simulink model "case6"  (R2024b)
settings: Solver=FixedStepAuto  StartTime=0  StopTime=1  FixedStep=1e-7  RelTol=1e-3
values from neighbouring files (symbols this model uses):
  SG_D_1_D = 0.01056    [IEEE9_case_parameters.m]    (also in case1_parameters.m; case2_parameters.m; case3_parameters.m; case4_parameters.m)
  SG_D_1_EnableSaturation = 0    [IEEE9_case_parameters.m]    (also in case1_parameters.m; case2_parameters.m; case3_parameters.m; case4_parameters.m)
  SG_D_1_f0 = 60    [IEEE9_case_parameters.m]    (also in case1_parameters.m; case2_parameters.m; case3_parameters.m; case4_parameters.m)
  SG_D_1_H = 7.5    [IEEE9_case_parameters.m]    (also in case1_parameters.m; case2_parameters.m; case3_parameters.m; case4_parameters.m)
  SG_D_1_K_A = 20    [IEEE9_case_parameters.m]    (also in case1_parameters.m; case2_parameters.m; case3_parameters.m; case4_parameters.m)
  SG_D_1_K_E = 1.000000e+1    (= 10)    [IEEE9_case_parameters.m]    (also in case1_parameters.m; case2_parameters.m; case3_parameters.m; case4_parameters.m)
  SG_D_1_K_F = 2.363    [IEEE9_case_parameters.m]    (also in case1_parameters.m; case2_parameters.m; case3_parameters.m; case4_parameters.m)
  SG_D_1_K_s = 0.5    [IEEE9_case_parameters.m]    (also in case1_parameters.m = 5; case2_parameters.m = 5; case3_parameters.m = 5; case4_parameters.m = 5)
  SG_D_1_R_a = 0.001088    [IEEE9_case_parameters.m]    (also in case1_parameters.m; case2_parameters.m; case3_parameters.m; case4_parameters.m)
  SG_D_1_S_A = 1    [IEEE9_case_parameters.m]    (also in case1_parameters.m; case2_parameters.m; case3_parameters.m; case4_parameters.m)
  SG_D_1_S_B = 0.103    [IEEE9_case_parameters.m]    (also in case1_parameters.m; case2_parameters.m; case3_parameters.m; case4_parameters.m)
  SG_D_1_S_N = 10.659857    [IEEE9_case_parameters.m]    (also in case1_parameters.m; case2_parameters.m; case3_parameters.m; case4_parameters.m)
  SG_D_1_SpeedPara = 200    [IEEE9_case_parameters.m]    (also in case1_parameters.m; case2_parameters.m; case3_parameters.m; case4_parameters.m)
  SG_D_1_T_0 = 0.720173    [IEEE9_case_parameters.m]    (also in case1_parameters.m = 0.755522; case2_parameters.m = 0.808931; case3_parameters.m = 0.869402; case4_parameters.m = 0.729316)
  SG_D_1_T_1 = 0.3    [IEEE9_case_parameters.m]    (also in case1_parameters.m; case2_parameters.m; case3_parameters.m; case4_parameters.m)
  SG_D_1_T_2 = 0.05    [IEEE9_case_parameters.m]    (also in case1_parameters.m; case2_parameters.m; case3_parameters.m; case4_parameters.m)
  SG_D_1_T_3 = 0.02    [IEEE9_case_parameters.m]    (also in case1_parameters.m; case2_parameters.m; case3_parameters.m; case4_parameters.m)
  SG_D_1_T_4 = 0.005    [IEEE9_case_parameters.m]    (also in case1_parameters.m; case2_parameters.m; case3_parameters.m; case4_parameters.m)
  SG_D_1_T_A = 0.02    [IEEE9_case_parameters.m]    (also in case1_parameters.m; case2_parameters.m; case3_parameters.m; case4_parameters.m)
  SG_D_1_T_dd = 8.000000e+0    (= 8)    [IEEE9_case_parameters.m]    (also in case1_parameters.m; case2_parameters.m; case3_parameters.m; case4_parameters.m)
  SG_D_1_T_ddd = 0.04    [IEEE9_case_parameters.m]    (also in case1_parameters.m; case2_parameters.m; case3_parameters.m; case4_parameters.m)
  SG_D_1_T_E = 0.314    [IEEE9_case_parameters.m]    (also in case1_parameters.m; case2_parameters.m; case3_parameters.m; case4_parameters.m)
  SG_D_1_T_F = 0.35    [IEEE9_case_parameters.m]    (also in case1_parameters.m; case2_parameters.m; case3_parameters.m; case4_parameters.m)
  SG_D_1_T_qd = 0.8    [IEEE9_case_parameters.m]    (also in case1_parameters.m; case2_parameters.m; case3_parameters.m; case4_parameters.m)
  SG_D_1_T_qdd = 0.02    [IEEE9_case_parameters.m]    (also in case1_parameters.m; case2_parameters.m; case3_parameters.m; case4_parameters.m)
  SG_D_1_T_speed = 0.1    [IEEE9_case_parameters.m]    (also in case1_parameters.m = 200; case2_parameters.m = 200; case3_parameters.m = 200; case4_parameters.m = 200)
  SG_D_1_T_w = 0.5    [IEEE9_case_parameters.m]    (also in case1_parameters.m; case2_parameters.m; case3_parameters.m; case4_parameters.m)
  SG_D_1_V_ref = 1.990276    [IEEE9_case_parameters.m]    (also in case1_parameters.m = 2.042296; case2_parameters.m = 2.051388; case3_parameters.m = 2.089584; case4_parameters.m = 2.01845)
  SG_D_1_w_ref = 376.991118    [IEEE9_case_parameters.m]    (also in case1_parameters.m; case2_parameters.m; case3_parameters.m; case4_parameters.m)
  SG_D_1_wb = 6.000000e+1    (= 60)    [IEEE9_case_parameters.m]    (also in case1_parameters.m; case2_parameters.m; case3_parameters.m; case4_parameters.m)
  SG_D_1_x_d = 1.9    [IEEE9_case_parameters.m]    (also in case1_parameters.m; case2_parameters.m; case3_parameters.m; case4_parameters.m)
  SG_D_1_x_dd = 0.302    [IEEE9_case_parameters.m]    (also in case1_parameters.m; case2_parameters.m; case3_parameters.m; case4_parameters.m)
  SG_D_1_x_ddd = 0.204    [IEEE9_case_parameters.m]    (also in case1_parameters.m; case2_parameters.m; case3_parameters.m; case4_parameters.m)
  SG_D_1_x_l = 0.05    [IEEE9_case_parameters.m]    (also in case1_parameters.m; case2_parameters.m; case3_parameters.m; case4_parameters.m)
  SG_D_1_x_q = 1.3    [IEEE9_case_parameters.m]    (also in case1_parameters.m; case2_parameters.m; case3_parameters.m; case4_parameters.m)
  SG_D_1_x_qd = 0.5    [IEEE9_case_parameters.m]    (also in case1_parameters.m; case2_parameters.m; case3_parameters.m; case4_parameters.m)
  SG_D_1_x_qdd = 0.3    [IEEE9_case_parameters.m]    (also in case1_parameters.m; case2_parameters.m; case3_parameters.m; case4_parameters.m)
  SG_D_2_D = 0.02    [IEEE9_case_parameters.m]    (also in case1_parameters.m; case2_parameters.m; case3_parameters.m; case4_parameters.m)
  SG_D_2_EnableSaturation = 0    [IEEE9_case_parameters.m]    (also in case1_parameters.m; case2_parameters.m; case3_parameters.m; case4_parameters.m)
  SG_D_2_f0 = 60    [IEEE9_case_parameters.m]    (also in case1_parameters.m; case2_parameters.m; case3_parameters.m; case4_parameters.m)
  SG_D_2_H = 8.000000e+0    (= 8)    [IEEE9_case_parameters.m]    (also in case1_parameters.m; case2_parameters.m; case3_parameters.m; case4_parameters.m)
  SG_D_2_K_A = 20    [IEEE9_case_parameters.m]    (also in case1_parameters.m; case2_parameters.m; case3_parameters.m; case4_parameters.m)
  SG_D_2_K_E = 1.000000e+1    (= 10)    [IEEE9_case_parameters.m]    (also in case1_parameters.m; case2_parameters.m; case3_parameters.m; case4_parameters.m)
  SG_D_2_K_F = 2.363    [IEEE9_case_parameters.m]    (also in case1_parameters.m; case2_parameters.m; case3_parameters.m; case4_parameters.m)
  SG_D_2_K_s = 0.5    [IEEE9_case_parameters.m]    (also in case1_parameters.m = 4; case2_parameters.m = 4; case3_parameters.m = 4; case4_parameters.m = 4)
  SG_D_2_R_a = 0.001088    [IEEE9_case_parameters.m]    (also in case1_parameters.m; case2_parameters.m; case3_parameters.m; case4_parameters.m)
  SG_D_2_S_A = 1    [IEEE9_case_parameters.m]    (also in case1_parameters.m; case2_parameters.m; case3_parameters.m; case4_parameters.m)
  SG_D_2_S_B = 0.103    [IEEE9_case_parameters.m]    (also in case1_parameters.m; case2_parameters.m; case3_parameters.m; case4_parameters.m)
  SG_D_2_S_N = 10.659857    [IEEE9_case_parameters.m]    (also in case1_parameters.m; case2_parameters.m; case3_parameters.m; case4_parameters.m)
  SG_D_2_SpeedPara = 200    [IEEE9_case_parameters.m]    (also in case1_parameters.m; case2_parameters.m; case3_parameters.m; case4_parameters.m)
  SG_D_2_T_0 = 1.632913    [IEEE9_case_parameters.m]    (also in case1_parameters.m = 1.632925; case2_parameters.m = 1.632915; case3_parameters.m = 1.632914; case4_parameters.m = 1.632927)
  SG_D_2_T_1 = 0.2    [IEEE9_case_parameters.m]    (also in case1_parameters.m; case2_parameters.m; case3_parameters.m; case4_parameters.m)
  SG_D_2_T_2 = 0.05    [IEEE9_case_parameters.m]    (also in case1_parameters.m; case2_parameters.m; case3_parameters.m; case4_parameters.m)
  SG_D_2_T_3 = 0.02    [IEEE9_case_parameters.m]    (also in case1_parameters.m; case2_parameters.m; case3_parameters.m; case4_parameters.m)
  SG_D_2_T_4 = 0.005    [IEEE9_case_parameters.m]    (also in case1_parameters.m; case2_parameters.m; case3_parameters.m; case4_parameters.m)
  SG_D_2_T_A = 0.02    [IEEE9_case_parameters.m]    (also in case1_parameters.m; case2_parameters.m; case3_parameters.m; case4_parameters.m)
  SG_D_2_T_dd = 7.9    [IEEE9_case_parameters.m]    (also in case1_parameters.m; case2_parameters.m; case3_parameters.m; case4_parameters.m)
  SG_D_2_T_ddd = 0.04    [IEEE9_case_parameters.m]    (also in case1_parameters.m; case2_parameters.m; case3_parameters.m; case4_parameters.m)
  SG_D_2_T_E = 0.314    [IEEE9_case_parameters.m]    (also in case1_parameters.m; case2_parameters.m; case3_parameters.m; case4_parameters.m)
  SG_D_2_T_F = 0.35    [IEEE9_case_parameters.m]    (also in case1_parameters.m; case2_parameters.m; case3_parameters.m; case4_parameters.m)
  SG_D_2_T_qd = 0.8    [IEEE9_case_parameters.m]    (also in case1_parameters.m; case2_parameters.m; case3_parameters.m; case4_parameters.m)
  SG_D_2_T_qdd = 0.015    [IEEE9_case_parameters.m]    (also in case1_parameters.m; case2_parameters.m; case3_parameters.m; case4_parameters.m)
  SG_D_2_T_speed = 0.1    [IEEE9_case_parameters.m]    (also in case1_parameters.m = 150; case2_parameters.m = 150; case3_parameters.m = 150; case4_parameters.m = 150)
  SG_D_2_T_w = 0.35    [IEEE9_case_parameters.m]    (also in case1_parameters.m; case2_parameters.m; case3_parameters.m; case4_parameters.m)
  SG_D_2_V_ref = 2.58547    [IEEE9_case_parameters.m]    (also in case1_parameters.m = 2.597896; case2_parameters.m = 2.587136; case3_parameters.m = 2.586042; case4_parameters.m = 2.599679)
  SG_D_2_w_ref = 376.991118    [IEEE9_case_parameters.m]    (also in case1_parameters.m; case2_parameters.m; case3_parameters.m; case4_parameters.m)
  SG_D_2_wb = 6.000000e+1    (= 60)    [IEEE9_case_parameters.m]    (also in case1_parameters.m; case2_parameters.m; case3_parameters.m; case4_parameters.m)
  SG_D_2_x_d = 1.8    [IEEE9_case_parameters.m]    (also in case1_parameters.m; case2_parameters.m; case3_parameters.m; case4_parameters.m)
  SG_D_2_x_dd = 0.302    [IEEE9_case_parameters.m]    (also in case1_parameters.m; case2_parameters.m; case3_parameters.m; case4_parameters.m)
  SG_D_2_x_ddd = 0.204    [IEEE9_case_parameters.m]    (also in case1_parameters.m; case2_parameters.m; case3_parameters.m; case4_parameters.m)
  SG_D_2_x_l = 0.05    [IEEE9_case_parameters.m]    (also in case1_parameters.m; case2_parameters.m; case3_parameters.m; case4_parameters.m)
  SG_D_2_x_q = 1.25    [IEEE9_case_parameters.m]    (also in case1_parameters.m; case2_parameters.m; case3_parameters.m; case4_parameters.m)
  SG_D_2_x_qd = 0.5    [IEEE9_case_parameters.m]    (also in case1_parameters.m; case2_parameters.m; case3_parameters.m; case4_parameters.m)
  SG_D_2_x_qdd = 0.3    [IEEE9_case_parameters.m]    (also in case1_parameters.m; case2_parameters.m; case3_parameters.m; case4_parameters.m)
  SG_D_3_D = 0.02    [IEEE9_case_parameters.m]    (also in case1_parameters.m; case2_parameters.m; case3_parameters.m; case4_parameters.m)
  SG_D_3_EnableSaturation = 0    [IEEE9_case_parameters.m]    (also in case1_parameters.m; case2_parameters.m; case3_parameters.m; case4_parameters.m)
  SG_D_3_f0 = 60    [IEEE9_case_parameters.m]    (also in case1_parameters.m; case2_parameters.m; case3_parameters.m; case4_parameters.m)
  SG_D_3_H = 7.7    [IEEE9_case_parameters.m]    (also in case1_parameters.m; case2_parameters.m; case3_parameters.m; case4_parameters.m)
  SG_D_3_K_A = 20    [IEEE9_case_parameters.m]    (also in case1_parameters.m; case2_parameters.m; case3_parameters.m; case4_parameters.m)
  SG_D_3_K_E = 1.000000e+1    (= 10)    [IEEE9_case_parameters.m]    (also in case1_parameters.m; case2_parameters.m; case3_parameters.m; case4_parameters.m)
  SG_D_3_K_F = 2.363    [IEEE9_case_parameters.m]    (also in case1_parameters.m; case2_parameters.m; case3_parameters.m; case4_parameters.m)
  SG_D_3_K_s = 0.2    [IEEE9_case_parameters.m]    (also in case1_parameters.m = 2; case2_parameters.m = 2; case3_parameters.m = 2; case4_parameters.m = 2)
  SG_D_3_R_a = 0.001088    [IEEE9_case_parameters.m]    (also in case1_parameters.m; case2_parameters.m; case3_parameters.m; case4_parameters.m)
  SG_D_3_S_A = 1    [IEEE9_case_parameters.m]    (also in case1_parameters.m; case2_parameters.m; case3_parameters.m; case4_parameters.m)
  SG_D_3_S_B = 0.103    [IEEE9_case_parameters.m]    (also in case1_parameters.m; case2_parameters.m; case3_parameters.m; case4_parameters.m)
  SG_D_3_S_N = 10.659857    [IEEE9_case_parameters.m]    (also in case1_parameters.m; case2_parameters.m; case3_parameters.m; case4_parameters.m)
  SG_D_3_SpeedPara = 200    [IEEE9_case_parameters.m]    (also in case1_parameters.m; case2_parameters.m; case3_parameters.m; case4_parameters.m)
  SG_D_3_T_0 = 0.850788    [IEEE9_case_parameters.m]    (also in case1_parameters.m = 0.850786; case2_parameters.m = 0.850787; case3_parameters.m; case4_parameters.m = 0.850786)
  SG_D_3_T_1 = 0.2    [IEEE9_case_parameters.m]    (also in case1_parameters.m; case2_parameters.m; case3_parameters.m; case4_parameters.m)
  SG_D_3_T_2 = 0.05    [IEEE9_case_parameters.m]    (also in case1_parameters.m; case2_parameters.m; case3_parameters.m; case4_parameters.m)
  SG_D_3_T_3 = 0.02    [IEEE9_case_parameters.m]    (also in case1_parameters.m; case2_parameters.m; case3_parameters.m; case4_parameters.m)
  SG_D_3_T_4 = 0.005    [IEEE9_case_parameters.m]    (also in case1_parameters.m; case2_parameters.m; case3_parameters.m; case4_parameters.m)
  SG_D_3_T_A = 0.02    [IEEE9_case_parameters.m]    (also in case1_parameters.m; case2_parameters.m; case3_parameters.m; case4_parameters.m)
  SG_D_3_T_dd = 8.1    [IEEE9_case_parameters.m]    (also in case1_parameters.m; case2_parameters.m; case3_parameters.m; case4_parameters.m)
  SG_D_3_T_ddd = 0.04    [IEEE9_case_parameters.m]    (also in case1_parameters.m; case2_parameters.m; case3_parameters.m; case4_parameters.m)
  SG_D_3_T_E = 0.314    [IEEE9_case_parameters.m]    (also in case1_parameters.m; case2_parameters.m; case3_parameters.m; case4_parameters.m)
  SG_D_3_T_F = 0.35    [IEEE9_case_parameters.m]    (also in case1_parameters.m; case2_parameters.m; case3_parameters.m; case4_parameters.m)
  SG_D_3_T_qd = 0.8    [IEEE9_case_parameters.m]    (also in case1_parameters.m; case2_parameters.m; case3_parameters.m; case4_parameters.m)
  SG_D_3_T_qdd = 0.015    [IEEE9_case_parameters.m]    (also in case1_parameters.m; case2_parameters.m; case3_parameters.m; case4_parameters.m)
  SG_D_3_T_speed = 0.1    [IEEE9_case_parameters.m]    (also in case1_parameters.m = 180; case2_parameters.m = 180; case3_parameters.m = 180; case4_parameters.m = 180)
  SG_D_3_T_w = 0.4    [IEEE9_case_parameters.m]    (also in case1_parameters.m; case2_parameters.m; case3_parameters.m; case4_parameters.m)
  SG_D_3_V_ref = 1.892727    [IEEE9_case_parameters.m]    (also in case1_parameters.m = 1.906439; case2_parameters.m = 1.895535; case3_parameters.m = 1.892105; case4_parameters.m = 1.906598)
  SG_D_3_w_ref = 376.991118    [IEEE9_case_parameters.m]    (also in case1_parameters.m; case2_parameters.m; case3_parameters.m; case4_parameters.m)
  SG_D_3_wb = 6.000000e+1    (= 60)    [IEEE9_case_parameters.m]    (also in case1_parameters.m; case2_parameters.m; case3_parameters.m; case4_parameters.m)
  SG_D_3_x_d = 1.85    [IEEE9_case_parameters.m]    (also in case1_parameters.m; case2_parameters.m; case3_parameters.m; case4_parameters.m)
  SG_D_3_x_dd = 0.302    [IEEE9_case_parameters.m]    (also in case1_parameters.m; case2_parameters.m; case3_parameters.m; case4_parameters.m)
  SG_D_3_x_ddd = 0.204    [IEEE9_case_parameters.m]    (also in case1_parameters.m; case2_parameters.m; case3_parameters.m; case4_parameters.m)
  SG_D_3_x_l = 0.05    [IEEE9_case_parameters.m]    (also in case1_parameters.m; case2_parameters.m; case3_parameters.m; case4_parameters.m)
  SG_D_3_x_q = 1.2    [IEEE9_case_parameters.m]    (also in case1_parameters.m; case2_parameters.m; case3_parameters.m; case4_parameters.m)
  SG_D_3_x_qd = 0.5    [IEEE9_case_parameters.m]    (also in case1_parameters.m; case2_parameters.m; case3_parameters.m; case4_parameters.m)
  SG_D_3_x_qdd = 0.3    [IEEE9_case_parameters.m]    (also in case1_parameters.m; case2_parameters.m; case3_parameters.m; case4_parameters.m)
(part 1 of 12)
settings Model: Creator=Greg  LastModifiedBy=Greg

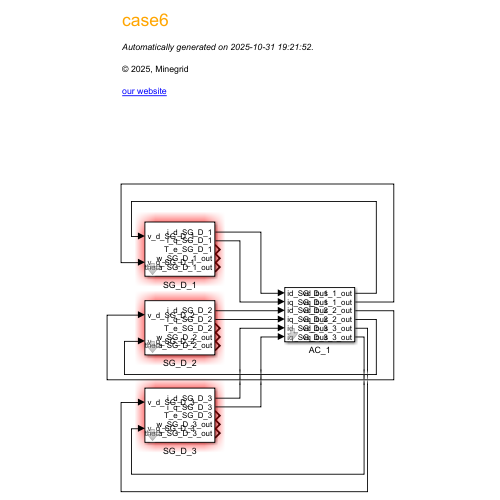
[thumbnail: Simulink's stored preview of the top-level diagram]
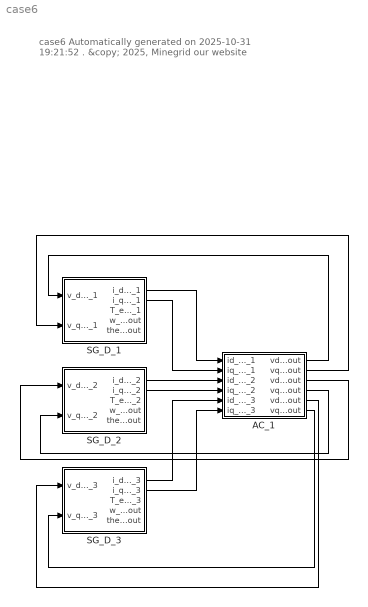
== system case6 ==
  note: case6
      | Automatically generated on 2025-10-31 19:21:52 .
      | &copy; 2025, Minegrid
      | our website
  AC_1 : Subsystem  mask(AC_1){}
      mask help: Parameters Interface of AC_1
  SG_D_1 : Subsystem  mask(SG_D_1){T_0=SG_D_1_T_0, w_ref=SG_D_1_w_ref, V_ref=SG_D_1_V_ref, x_d=SG_D_1_x_d, x_dd=SG_D_1_x_dd, x_ddd=SG_D_1_x_ddd, x_q=SG_D_1_x_q, x_qd=SG_D_1_x_qd, x_qdd=SG_D_1_x_qdd, x_l=SG_D_1_x_l, R_a=SG_D_1_R_a, T_dd=SG_D_1_T_dd, T_ddd=SG_D_1_T_ddd, T_qd=SG_D_1_T_qd, T_qdd=SG_D_1_T_qdd, H=SG_D_1_H, D=SG_D_1_D, SpeedPara=SG_D_1_SpeedPara, K_A=SG_D_1_K_A, EnableSaturation=SG_D_1_EnableSaturation, f0=SG_D_1_f0, T_speed=SG_D_1_T_speed, T_E=SG_D_1_T_E, T_A=SG_D_1_T_A, T_F=SG_D_1_T_F, K_E=SG_D_1_K_E, K_F=SG_D_1_K_F, K_s=SG_D_1_K_s, T_1=SG_D_1_T_1, T_2=SG_D_1_T_2, T_3=SG_D_1_T_3, T_4=SG_D_1_T_4, T_w=SG_D_1_T_w, wb=SG_D_1_wb, S_A=SG_D_1_S_A, S_B=SG_D_1_S_B, S_N=SG_D_1_S_N}
      mask help: Parameters Interface of SG_D_1
  SG_D_2 : Subsystem  mask(SG_D_2){T_0=SG_D_2_T_0, w_ref=SG_D_2_w_ref, V_ref=SG_D_2_V_ref, x_d=SG_D_2_x_d, x_dd=SG_D_2_x_dd, x_ddd=SG_D_2_x_ddd, x_q=SG_D_2_x_q, x_qd=SG_D_2_x_qd, x_qdd=SG_D_2_x_qdd, x_l=SG_D_2_x_l, R_a=SG_D_2_R_a, T_dd=SG_D_2_T_dd, T_ddd=SG_D_2_T_ddd, T_qd=SG_D_2_T_qd, T_qdd=SG_D_2_T_qdd, H=SG_D_2_H, D=SG_D_2_D, SpeedPara=SG_D_2_SpeedPara, K_A=SG_D_2_K_A, EnableSaturation=SG_D_2_EnableSaturation, f0=SG_D_2_f0, T_speed=SG_D_2_T_speed, T_E=SG_D_2_T_E, T_A=SG_D_2_T_A, T_F=SG_D_2_T_F, K_E=SG_D_2_K_E, K_F=SG_D_2_K_F, K_s=SG_D_2_K_s, T_1=SG_D_2_T_1, T_2=SG_D_2_T_2, T_3=SG_D_2_T_3, T_4=SG_D_2_T_4, T_w=SG_D_2_T_w, wb=SG_D_2_wb, S_A=SG_D_2_S_A, S_B=SG_D_2_S_B, S_N=SG_D_2_S_N}
      mask help: Parameters Interface of SG_D_2
  SG_D_3 : Subsystem  mask(SG_D_3){T_0=SG_D_3_T_0, w_ref=SG_D_3_w_ref, V_ref=SG_D_3_V_ref, x_d=SG_D_3_x_d, x_dd=SG_D_3_x_dd, x_ddd=SG_D_3_x_ddd, x_q=SG_D_3_x_q, x_qd=SG_D_3_x_qd, x_qdd=SG_D_3_x_qdd, x_l=SG_D_3_x_l, R_a=SG_D_3_R_a, T_dd=SG_D_3_T_dd, T_ddd=SG_D_3_T_ddd, T_qd=SG_D_3_T_qd, T_qdd=SG_D_3_T_qdd, H=SG_D_3_H, D=SG_D_3_D, SpeedPara=SG_D_3_SpeedPara, K_A=SG_D_3_K_A, EnableSaturation=SG_D_3_EnableSaturation, f0=SG_D_3_f0, T_speed=SG_D_3_T_speed, T_E=SG_D_3_T_E, T_A=SG_D_3_T_A, T_F=SG_D_3_T_F, K_E=SG_D_3_K_E, K_F=SG_D_3_K_F, K_s=SG_D_3_K_s, T_1=SG_D_3_T_1, T_2=SG_D_3_T_2, T_3=SG_D_3_T_3, T_4=SG_D_3_T_4, T_w=SG_D_3_T_w, wb=SG_D_3_wb, S_A=SG_D_3_S_A, S_B=SG_D_3_S_B, S_N=SG_D_3_S_N}
      mask help: Parameters Interface of SG_D_3
  wires:
  SG_D_2/2(i_q_SG_D_2) -> AC_1/4(iq_SG_D_2)
  SG_D_1/2(i_q_SG_D_1) -> AC_1/2(iq_SG_D_1)
  SG_D_1/1(i_d_SG_D_1) -> AC_1/1(id_SG_D_1)
  SG_D_2/1(i_d_SG_D_2) -> AC_1/3(id_SG_D_2)
  AC_1/1(vd_bus_1_out) -> SG_D_1/1(v_d_SG_D_1)
  SG_D_3/1(i_d_SG_D_3) -> AC_1/5(id_SG_D_3)
  AC_1/2(vq_bus_1_out) -> SG_D_1/2(v_q_SG_D_1)
  SG_D_3/2(i_q_SG_D_3) -> AC_1/6(iq_SG_D_3)
  AC_1/3(vd_bus_2_out) -> SG_D_2/1(v_d_SG_D_2)
  AC_1/4(vq_bus_2_out) -> SG_D_2/2(v_q_SG_D_2)
  AC_1/5(vd_bus_3_out) -> SG_D_3/1(v_d_SG_D_3)
  AC_1/6(vq_bus_3_out) -> SG_D_3/2(v_q_SG_D_3)

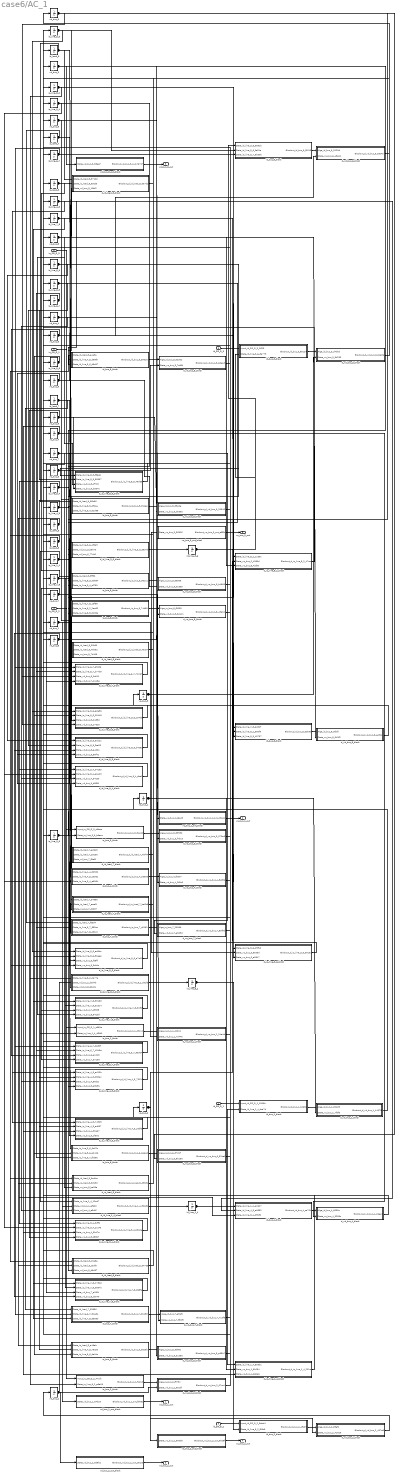
== system case6/AC_1 ==
  id_SG_D_1 : Inport
  iq_SG_D_1 : Inport  Port=2
  id_SG_D_2 : Inport  Port=3
  iq_SG_D_2 : Inport  Port=4
  id_SG_D_3 : Inport  Port=5
  iq_SG_D_3 : Inport  Port=6
  d_id_line_1_4_block : Subsystem
  d_id_line_3_6_block : Subsystem
  d_id_line_4_5_block : Subsystem
  d_id_line_5_6_block : Subsystem
  d_id_line_6_7_block : Subsystem
  d_id_line_7_8_block : Subsystem
  d_id_line_8_2_block : Subsystem
  d_id_line_8_9_block : Subsystem
  d_id_line_9_4_block : Subsystem
  d_id_load_5_block : Subsystem
  d_id_load_7_block : Subsystem
  d_id_load_9_block : Subsystem
  d_iq_line_1_4_block : Subsystem
  d_iq_line_3_6_block : Subsystem
  d_iq_line_4_5_block : Subsystem
  d_iq_line_5_6_block : Subsystem
  d_iq_line_6_7_block : Subsystem
  d_iq_line_7_8_block : Subsystem
  d_iq_line_8_2_block : Subsystem
  d_iq_line_8_9_block : Subsystem
  d_iq_line_9_4_block : Subsystem
  d_iq_load_5_block : Subsystem
  d_iq_load_7_block : Subsystem
  d_iq_load_9_block : Subsystem
  d_vd_bus_1_block : Subsystem
  d_vd_bus_2_block : Subsystem
  d_vd_bus_3_block : Subsystem
  d_vd_bus_4_block : Subsystem
  d_vd_bus_5_block : Subsystem
  d_vd_bus_6_block : Subsystem
  d_vd_bus_7_block : Subsystem
  d_vd_bus_8_block : Subsystem
  d_vd_bus_9_block : Subsystem
  d_vq_bus_1_block : Subsystem
  d_vq_bus_2_block : Subsystem
  d_vq_bus_3_block : Subsystem
  d_vq_bus_4_block : Subsystem
  d_vq_bus_5_block : Subsystem
  d_vq_bus_6_block : Subsystem
  d_vq_bus_7_block : Subsystem
  d_vq_bus_8_block : Subsystem
  d_vq_bus_9_block : Subsystem
  id_bus_1_block : Subsystem
  id_bus_2_block : Subsystem
  id_bus_3_block : Subsystem
  id_bus_4_block : Subsystem
  id_bus_5_block : Subsystem
  id_bus_6_block : Subsystem
  id_bus_7_block : Subsystem
  id_bus_8_block : Subsystem
  id_bus_9_block : Subsystem
  id_line_1_4 : Integrator  InitialCondition=0.6234
  id_line_3_6 : Integrator  InitialCondition=0.8417
  id_line_4_5 : Integrator  InitialCondition=0.2653
  id_line_5_6 : Integrator  InitialCondition=-0.6233
  id_line_6_7 : Integrator  InitialCondition=0.231
  id_line_7_8 : Integrator  InitialCondition=-0.7536
  id_line_8_2 : Integrator  InitialCondition=-1.626
  id_line_8_9 : Integrator  InitialCondition=0.8896
  id_line_9_4 : Integrator  InitialCondition=-0.3524
  id_load_5 : Integrator  InitialCondition=0.874158966299017
  id_load_7 : Integrator  InitialCondition=0.9889641534008289
  id_load_9 : Integrator  InitialCondition=1.227763176441315
  iq_bus_1_block : Subsystem
  iq_bus_2_block : Subsystem
  iq_bus_3_block : Subsystem
  iq_bus_4_block : Subsystem
  iq_bus_5_block : Subsystem
  iq_bus_6_block : Subsystem
  iq_bus_7_block : Subsystem
  iq_bus_8_block : Subsystem
  iq_bus_9_block : Subsystem
  iq_line_1_4 : Integrator  InitialCondition=-0.247
  iq_line_3_6 : Integrator  InitialCondition=0.129
  iq_line_4_5 : Integrator  InitialCondition=-0.0899
  iq_line_5_6 : Integrator  InitialCondition=0.0171
  iq_line_6_7 : Integrator  InitialCondition=-0.1383
  iq_line_7_8 : Integrator  InitialCondition=0.0156
  iq_line_8_2 : Integrator  InitialCondition=-0.1643
  iq_line_8_9 : Integrator  InitialCondition=-0.0464
  iq_line_9_4 : Integrator  InitialCondition=0.3218
  iq_load_5 : Integrator  InitialCondition=-0.35817674392091936
  iq_load_7 : Integrator  InitialCondition=-0.3305459238036955
  iq_load_9 : Integrator  InitialCondition=-0.5986873382546184
  vd_bus_1 : Integrator  InitialCondition=1.0
  vd_bus_1_out_block : Subsystem
  vd_bus_2 : Integrator  InitialCondition=0.9850168221162429
  vd_bus_2_out_block : Subsystem
  vd_bus_3 : Integrator  InitialCondition=0.9958098670951172
  vd_bus_3_out_block : Subsystem
  vd_bus_4 : Integrator  InitialCondition=0.9864442922045917
  vd_bus_5 : Integrator  InitialCondition=0.9736252032903118
  vd_bus_6 : Integrator  InitialCondition=1.0030118698879946
  vd_bus_7 : Integrator  InitialCondition=0.986717281277157
  vd_bus_8 : Integrator  InitialCondition=0.9948040848836197
  vd_bus_9 : Integrator  InitialCondition=0.9565190377448524
  vq_bus_1 : Integrator  InitialCondition=0.0
  vq_bus_1_out_block : Subsystem
  vq_bus_2 : Integrator  InitialCondition=0.1724582852402808
  vq_bus_2_out_block : Subsystem
  vq_bus_3 : Integrator  InitialCondition=0.09144784631693036
  vq_bus_3_out_block : Subsystem
  vq_bus_4 : Integrator  InitialCondition=-0.03421786740856599
  vq_bus_5 : Integrator  InitialCondition=-0.055798679753154154
  vq_bus_6 : Integrator  InitialCondition=0.04444454431260476
  vq_bus_7 : Integrator  InitialCondition=0.024055248459070585
  vq_bus_8 : Integrator  InitialCondition=0.07561642616061612
  vq_bus_9 : Integrator  InitialCondition=-0.05924122012533022
  vd_bus_1_out : Outport
  vq_bus_1_out : Outport  Port=2
  vd_bus_2_out : Outport  Port=3
  vq_bus_2_out : Outport  Port=4
  vd_bus_3_out : Outport  Port=5
  vq_bus_3_out : Outport  Port=6
  wires:
  vq_bus_2_out_block/1(Blockout_vq_bus_2_out_9bd8f) -> vq_bus_2_out/1
  d_id_line_1_4_block/1(Blockout_d_id_line_1_4_9b681) -> id_line_1_4/1
  iq_SG_D_3/1 -> iq_bus_3_block/1(Input_iq_SG_D_3_c9bea)
  id_SG_D_3/1 -> id_bus_3_block/1(Input_id_SG_D_3_f42f9)
  d_iq_line_8_2_block/1(Blockout_d_iq_line_8_2_47ccc) -> iq_line_8_2/1
  d_vd_bus_4_block/1(Blockout_d_vd_bus_4_26ea1) -> vd_bus_4/1
  vd_bus_3_out_block/1(Blockout_vd_bus_3_out_76727) -> vd_bus_3_out/1
  d_iq_load_7_block/1(Blockout_d_iq_load_7_ba6b6) -> iq_load_7/1
  id_SG_D_1/1 -> id_bus_1_block/1(Input_id_SG_D_1_1909b)
  id_SG_D_2/1 -> id_bus_2_block/1(Input_id_SG_D_2_3ebd4)
  d_id_line_4_5_block/1(Blockout_d_id_line_4_5_7311f) -> id_line_4_5/1
  id_line_8_2/1 -> d_iq_line_8_2_block/1(State_id_line_8_2_11e9c), id_bus_2_block/2(State_id_line_8_2_f66c5), id_bus_8_block/2(State_id_line_8_2_e60f9)
  iq_SG_D_2/1 -> iq_bus_2_block/1(Input_iq_SG_D_2_471fc)
  d_id_line_8_2_block/1(Blockout_d_id_line_8_2_da1fe) -> id_line_8_2/1
  d_id_line_7_8_block/1(Blockout_d_id_line_7_8_868fa) -> id_line_7_8/1
  id_bus_9_block/1(Blockout_id_bus_9_51cea) -> d_vd_bus_9_block/1(Alge_id_bus_9_39a0e)
  iq_SG_D_1/1 -> iq_bus_1_block/1(Input_iq_SG_D_1_c869a)
  iq_bus_9_block/1(Blockout_iq_bus_9_9e11c) -> d_vq_bus_9_block/1(Alge_iq_bus_9_635a6)
  vd_bus_2_out_block/1(Blockout_vd_bus_2_out_c0c26) -> vd_bus_2_out/1
  d_iq_line_7_8_block/1(Blockout_d_iq_line_7_8_31fbf) -> iq_line_7_8/1
  id_line_8_9/1 -> id_bus_8_block/3(State_id_line_8_9_45767), d_id_line_8_9_block/1(State_id_line_8_9_91b21), id_bus_9_block/2(State_id_line_8_9_df04e), d_iq_line_8_9_block/1(State_id_line_8_9_f86eb)
  vd_bus_3/1 -> d_vq_bus_3_block/2(State_vd_bus_3_f7b1a), d_id_line_3_6_block/2(State_vd_bus_3_b5b7a), vd_bus_3_out_block/1(State_vd_bus_3_58eaf)
  iq_line_9_4/1 -> d_id_line_9_4_block/2(State_iq_line_9_4_a6420), d_iq_line_9_4_block/2(State_iq_line_9_4_21c4a), iq_bus_4_block/3(State_iq_line_9_4_e6964), iq_bus_9_block/3(State_iq_line_9_4_af760)
  vq_bus_6/1 -> d_iq_line_3_6_block/3(State_vq_bus_6_e5847), d_vd_bus_6_block/2(State_vq_bus_6_48ab1), d_iq_line_6_7_block/3(State_vq_bus_6_e12d0), d_iq_line_5_6_block/4(State_vq_bus_6_9dc1c)
  d_iq_line_4_5_block/1(Blockout_d_iq_line_4_5_20bf0) -> iq_line_4_5/1
  vd_bus_8/1 -> d_vq_bus_8_block/2(State_vd_bus_8_bd411), d_id_line_7_8_block/4(State_vd_bus_8_cba40), d_id_line_8_9_block/3(State_vd_bus_8_64db1), d_id_line_8_2_block/3(State_vd_bus_8_6bcd4)
  vq_bus_3_out_block/1(Blockout_vq_bus_3_out_eff6b) -> vq_bus_3_out/1
  iq_bus_8_block/1(Blockout_iq_bus_8_74d80) -> d_vq_bus_8_block/1(Alge_iq_bus_8_f5035)
  id_bus_3_block/1(Blockout_id_bus_3_89124) -> d_vd_bus_3_block/1(Alge_id_bus_3_d4dbd)
  id_bus_8_block/1(Blockout_id_bus_8_eda9d) -> d_vd_bus_8_block/1(Alge_id_bus_8_0f2fd)
  vq_bus_1_out_block/1(Blockout_vq_bus_1_out_454ab) -> vq_bus_1_out/1
  vd_bus_1_out_block/1(Blockout_vd_bus_1_out_fd68c) -> vd_bus_1_out/1
  id_bus_4_block/1(Blockout_id_bus_4_ca704) -> d_vd_bus_4_block/1(Alge_id_bus_4_6035c)
  id_bus_6_block/1(Blockout_id_bus_6_f0019) -> d_vd_bus_6_block/1(Alge_id_bus_6_9129d)
  id_line_4_5/1 -> id_bus_4_block/2(State_id_line_4_5_a6682), d_iq_line_4_5_block/1(State_id_line_4_5_745b5), id_bus_5_block/2(State_id_line_4_5_d68f5), d_id_line_4_5_block/1(State_id_line_4_5_ad13b)
  iq_bus_7_block/1(Blockout_iq_bus_7_c0161) -> d_vq_bus_7_block/1(Alge_iq_bus_7_2005b)
  iq_bus_3_block/1(Blockout_iq_bus_3_54a2d) -> d_vq_bus_3_block/1(Alge_iq_bus_3_53990)
  id_load_5/1 -> d_iq_load_5_block/1(State_id_load_5_9ad4e), id_bus_5_block/1(State_id_load_5_e4a9a), d_id_load_5_block/1(State_id_load_5_13a8a)
  id_bus_7_block/1(Blockout_id_bus_7_0b458) -> d_vd_bus_7_block/1(Alge_id_bus_7_e9afc)
  vd_bus_9/1 -> d_vq_bus_9_block/2(State_vd_bus_9_01655), d_id_line_8_9_block/4(State_vd_bus_9_80f42), d_id_line_9_4_block/4(State_vd_bus_9_b5f80), d_id_load_9_block/3(State_vd_bus_9_1fdd2)
  d_vq_bus_2_block/1(Blockout_d_vq_bus_2_07cc4) -> vq_bus_2/1
  d_id_load_7_block/1(Blockout_d_id_load_7_4bf44) -> id_load_7/1
  iq_bus_6_block/1(Blockout_iq_bus_6_6aaed) -> d_vq_bus_6_block/1(Alge_iq_bus_6_37d1f)
  id_line_9_4/1 -> id_bus_4_block/3(State_id_line_9_4_09bfd), d_iq_line_9_4_block/1(State_id_line_9_4_3cff0), id_bus_9_block/3(State_id_line_9_4_02d88), d_id_line_9_4_block/1(State_id_line_9_4_0416a)
  d_iq_line_8_9_block/1(Blockout_d_iq_line_8_9_46de9) -> iq_line_8_9/1
  iq_load_5/1 -> d_id_load_5_block/2(State_iq_load_5_cadf3), iq_bus_5_block/1(State_iq_load_5_a48ab), d_iq_load_5_block/2(State_iq_load_5_32b90)
  id_line_6_7/1 -> id_bus_6_block/3(State_id_line_6_7_6b30b), d_id_line_6_7_block/1(State_id_line_6_7_65cd6), d_iq_line_6_7_block/1(State_id_line_6_7_b680f), id_bus_7_block/2(State_id_line_6_7_91e84)
  id_bus_2_block/1(Blockout_id_bus_2_4fb07) -> d_vd_bus_2_block/1(Alge_id_bus_2_89ef1)
  iq_bus_4_block/1(Blockout_iq_bus_4_aea66) -> d_vq_bus_4_block/1(Alge_iq_bus_4_f3ad7)
  iq_bus_2_block/1(Blockout_iq_bus_2_f1d15) -> d_vq_bus_2_block/1(Alge_iq_bus_2_f979c)
  vd_bus_6/1 -> d_vq_bus_6_block/2(State_vd_bus_6_8b156), d_id_line_3_6_block/3(State_vd_bus_6_77dc2), d_id_line_6_7_block/3(State_vd_bus_6_0c641), d_id_line_5_6_block/4(State_vd_bus_6_2762e)
  iq_bus_5_block/1(Blockout_iq_bus_5_b826b) -> d_vq_bus_5_block/1(Alge_iq_bus_5_9d80c)
  id_bus_5_block/1(Blockout_id_bus_5_39616) -> d_vd_bus_5_block/1(Alge_id_bus_5_023a2)
  iq_line_3_6/1 -> iq_bus_3_block/2(State_iq_line_3_6_b8aac), iq_bus_6_block/1(State_iq_line_3_6_6c42b), d_id_line_3_6_block/1(State_iq_line_3_6_1fda9)
  iq_bus_1_block/1(Blockout_iq_bus_1_c5112) -> d_vq_bus_1_block/1(Alge_iq_bus_1_c2b12)
  iq_line_7_8/1 -> d_id_line_7_8_block/2(State_iq_line_7_8_a857b), iq_bus_7_block/3(State_iq_line_7_8_c812c), iq_bus_8_block/1(State_iq_line_7_8_13f88), d_iq_line_7_8_block/2(State_iq_line_7_8_31614)
  id_line_3_6/1 -> id_bus_3_block/2(State_id_line_3_6_8a779), id_bus_6_block/1(State_id_line_3_6_9e91b), d_iq_line_3_6_block/1(State_id_line_3_6_29fbd)
  id_bus_1_block/1(Blockout_id_bus_1_b268c) -> d_vd_bus_1_block/1(Alge_id_bus_1_00dd9)
  d_iq_line_5_6_block/1(Blockout_d_iq_line_5_6_a7a19) -> iq_line_5_6/1
  id_load_7/1 -> d_iq_load_7_block/1(State_id_load_7_34556), id_bus_7_block/1(State_id_load_7_33856), d_id_load_7_block/1(State_id_load_7_ed6d0)
  vq_bus_4/1 -> d_vd_bus_4_block/2(State_vq_bus_4_3285c), d_iq_line_1_4_block/3(State_vq_bus_4_deba6), d_iq_line_9_4_block/3(State_vq_bus_4_9b47a), d_iq_line_4_5_block/3(State_vq_bus_4_3ba67)
  d_id_line_3_6_block/1(Blockout_d_id_line_3_6_6537b) -> id_line_3_6/1
  d_iq_load_5_block/1(Blockout_d_iq_load_5_d983c) -> iq_load_5/1
  d_id_line_5_6_block/1(Blockout_d_id_line_5_6_154da) -> id_line_5_6/1
  vq_bus_7/1 -> d_vd_bus_7_block/2(State_vq_bus_7_f5bf3), d_iq_load_7_block/3(State_vq_bus_7_dcb87), d_iq_line_7_8_block/3(State_vq_bus_7_c9505), d_iq_line_6_7_block/4(State_vq_bus_7_e72a8)
  vd_bus_4/1 -> d_id_line_1_4_block/3(State_vd_bus_4_e5c5f), d_id_line_4_5_block/3(State_vd_bus_4_56dcc), d_id_line_9_4_block/3(State_vd_bus_4_54ca0), d_vq_bus_4_block/2(State_vd_bus_4_f40b6)
  iq_line_8_9/1 -> d_id_line_8_9_block/2(State_iq_line_8_9_fbe05), d_iq_line_8_9_block/2(State_iq_line_8_9_58567), iq_bus_8_block/3(State_iq_line_8_9_0180a), iq_bus_9_block/2(State_iq_line_8_9_ad854)
  iq_line_8_2/1 -> d_id_line_8_2_block/1(State_iq_line_8_2_2a77a), iq_bus_2_block/2(State_iq_line_8_2_e8e09), iq_bus_8_block/2(State_iq_line_8_2_2ae52)
  vq_bus_9/1 -> d_iq_load_9_block/3(State_vq_bus_9_7d406), d_iq_line_8_9_block/4(State_vq_bus_9_b3e7a), d_iq_line_9_4_block/4(State_vq_bus_9_c88b7), d_vd_bus_9_block/2(State_vq_bus_9_da3ae)
  iq_load_7/1 -> d_id_load_7_block/2(State_iq_load_7_25236), d_iq_load_7_block/2(State_iq_load_7_eeef1), iq_bus_7_block/1(State_iq_load_7_fd394)
  id_line_7_8/1 -> id_bus_8_block/1(State_id_line_7_8_6dd2f), d_id_line_7_8_block/1(State_id_line_7_8_178dd), d_iq_line_7_8_block/1(State_id_line_7_8_93183), id_bus_7_block/3(State_id_line_7_8_65e8d)
  iq_line_6_7/1 -> d_id_line_6_7_block/2(State_iq_line_6_7_b77b9), d_iq_line_6_7_block/2(State_iq_line_6_7_4945e), iq_bus_6_block/3(State_iq_line_6_7_fbd66), iq_bus_7_block/2(State_iq_line_6_7_889cc)
  iq_line_1_4/1 -> d_id_line_1_4_block/1(State_iq_line_1_4_12ad7), iq_bus_1_block/2(State_iq_line_1_4_4f8d0), iq_bus_4_block/1(State_iq_line_1_4_0b9d2)
  vq_bus_1/1 -> vq_bus_1_out_block/1(State_vq_bus_1_c6ac3), d_iq_line_1_4_block/2(State_vq_bus_1_6b284), d_vd_bus_1_block/2(State_vq_bus_1_7fdf6)
  iq_line_5_6/1 -> d_id_line_5_6_block/2(State_iq_line_5_6_03448), d_iq_line_5_6_block/2(State_iq_line_5_6_5beea), iq_bus_5_block/3(State_iq_line_5_6_da04c), iq_bus_6_block/2(State_iq_line_5_6_a2426)
  id_line_5_6/1 -> id_bus_6_block/2(State_id_line_5_6_fe13e), d_id_line_5_6_block/1(State_id_line_5_6_ede96), d_iq_line_5_6_block/1(State_id_line_5_6_ed5dc), id_bus_5_block/3(State_id_line_5_6_d8d07)
  id_line_1_4/1 -> d_iq_line_1_4_block/1(State_id_line_1_4_5a9b1), id_bus_1_block/2(State_id_line_1_4_cba7d), id_bus_4_block/1(State_id_line_1_4_a2627)
  iq_line_4_5/1 -> d_id_line_4_5_block/2(State_iq_line_4_5_080ac), d_iq_line_4_5_block/2(State_iq_line_4_5_ac887), iq_bus_4_block/2(State_iq_line_4_5_235e1), iq_bus_5_block/2(State_iq_line_4_5_75c3a)
  vq_bus_2/1 -> d_iq_line_8_2_block/2(State_vq_bus_2_4380d), vq_bus_2_out_block/1(State_vq_bus_2_90ade), d_vd_bus_2_block/2(State_vq_bus_2_41626)
  iq_load_9/1 -> d_id_load_9_block/2(State_iq_load_9_63cda), d_iq_load_9_block/2(State_iq_load_9_4ab62), iq_bus_9_block/1(State_iq_load_9_3ff8b)
  id_load_9/1 -> d_id_load_9_block/1(State_id_load_9_971b0), d_iq_load_9_block/1(State_id_load_9_30bf6), id_bus_9_block/1(State_id_load_9_96b66)
  vq_bus_8/1 -> d_vd_bus_8_block/2(State_vq_bus_8_543f2), d_iq_line_8_2_block/3(State_vq_bus_8_42f30), d_iq_line_7_8_block/4(State_vq_bus_8_642dd), d_iq_line_8_9_block/3(State_vq_bus_8_cf718)
  vd_bus_7/1 -> d_vq_bus_7_block/2(State_vd_bus_7_eb09d), d_id_load_7_block/3(State_vd_bus_7_f8e0f), d_id_line_6_7_block/4(State_vd_bus_7_d448e), d_id_line_7_8_block/3(State_vd_bus_7_a03f4)
  vd_bus_5/1 -> d_vq_bus_5_block/2(State_vd_bus_5_a1a5e), d_id_load_5_block/3(State_vd_bus_5_d8d97), d_id_line_4_5_block/4(State_vd_bus_5_a3b9b), d_id_line_5_6_block/3(State_vd_bus_5_0485d)
  d_id_line_9_4_block/1(Blockout_d_id_line_9_4_cfcaf) -> id_line_9_4/1
  vq_bus_5/1 -> d_vd_bus_5_block/2(State_vq_bus_5_7e9fd), d_iq_load_5_block/3(State_vq_bus_5_ba55a), d_iq_line_4_5_block/4(State_vq_bus_5_1f302), d_iq_line_5_6_block/3(State_vq_bus_5_fd8ff)
  vq_bus_3/1 -> d_iq_line_3_6_block/2(State_vq_bus_3_8aa9d), d_vd_bus_3_block/2(State_vq_bus_3_8d253), vq_bus_3_out_block/1(State_vq_bus_3_38926)
  vd_bus_2/1 -> d_vq_bus_2_block/2(State_vd_bus_2_661bf), d_id_line_8_2_block/2(State_vd_bus_2_ddd4b), vd_bus_2_out_block/1(State_vd_bus_2_6d8b2)
  vd_bus_1/1 -> d_id_line_1_4_block/2(State_vd_bus_1_ef6b0), d_vq_bus_1_block/2(State_vd_bus_1_7d44a), vd_bus_1_out_block/1(State_vd_bus_1_64b20)
  d_iq_load_9_block/1(Blockout_d_iq_load_9_4ac07) -> iq_load_9/1
  d_vq_bus_1_block/1(Blockout_d_vq_bus_1_24e4d) -> vq_bus_1/1
  d_id_line_6_7_block/1(Blockout_d_id_line_6_7_71267) -> id_line_6_7/1
  d_vq_bus_3_block/1(Blockout_d_vq_bus_3_070a5) -> vq_bus_3/1
  d_id_line_8_9_block/1(Blockout_d_id_line_8_9_b4a61) -> id_line_8_9/1
  d_id_load_5_block/1(Blockout_d_id_load_5_e47ee) -> id_load_5/1
  d_id_load_9_block/1(Blockout_d_id_load_9_0a7d1) -> id_load_9/1
  d_vq_bus_8_block/1(Blockout_d_vq_bus_8_43ab1) -> vq_bus_8/1
  d_iq_line_1_4_block/1(Blockout_d_iq_line_1_4_201af) -> iq_line_1_4/1
  d_iq_line_3_6_block/1(Blockout_d_iq_line_3_6_a81a1) -> iq_line_3_6/1
  d_iq_line_6_7_block/1(Blockout_d_iq_line_6_7_9a304) -> iq_line_6_7/1
  d_vq_bus_5_block/1(Blockout_d_vq_bus_5_a65b7) -> vq_bus_5/1
  d_vq_bus_7_block/1(Blockout_d_vq_bus_7_5af5d) -> vq_bus_7/1
  d_vd_bus_1_block/1(Blockout_d_vd_bus_1_44375) -> vd_bus_1/1
  d_iq_line_9_4_block/1(Blockout_d_iq_line_9_4_b362e) -> iq_line_9_4/1
  d_vd_bus_2_block/1(Blockout_d_vd_bus_2_407e5) -> vd_bus_2/1
  d_vd_bus_3_block/1(Blockout_d_vd_bus_3_bca86) -> vd_bus_3/1
  d_vd_bus_9_block/1(Blockout_d_vd_bus_9_20840) -> vd_bus_9/1
  d_vd_bus_5_block/1(Blockout_d_vd_bus_5_60ea3) -> vd_bus_5/1
  d_vd_bus_6_block/1(Blockout_d_vd_bus_6_93c4a) -> vd_bus_6/1
  d_vd_bus_7_block/1(Blockout_d_vd_bus_7_71af8) -> vd_bus_7/1
  d_vd_bus_8_block/1(Blockout_d_vd_bus_8_ec3c4) -> vd_bus_8/1
  d_vq_bus_4_block/1(Blockout_d_vq_bus_4_5efd6) -> vq_bus_4/1
  d_vq_bus_6_block/1(Blockout_d_vq_bus_6_51bef) -> vq_bus_6/1
  d_vq_bus_9_block/1(Blockout_d_vq_bus_9_b4666) -> vq_bus_9/1

== system case6/SG_D_1 ==
  v_d_SG_D_1 : Inport
  v_q_SG_D_1 : Inport  Port=2
  E_fd_SG_D_1 : Integrator  InitialCondition=1.872088065832508
  Px_1_SG_D_1 : Integrator  InitialCondition=0.0
  Px_2_SG_D_1 : Integrator  InitialCondition=0.0
  Px_3_SG_D_1 : Integrator  InitialCondition=-2.4274939065845613e-29
  R_f_SG_D_1 : Integrator  InitialCondition=12.639268855892048
  T_e_SG_D_1_block : Subsystem
  T_m_SG_D_1 : Integrator  InitialCondition=0.6238993705978026
  V_f_SG_D_1 : Integrator  InitialCondition=18.72088065832508
  d_E_fd_SG_D_1_block : Subsystem
  d_Px_1_SG_D_1_block : Subsystem
  d_Px_2_SG_D_1_block : Subsystem
  d_Px_3_SG_D_1_block : Subsystem
  d_R_f_SG_D_1_block : Subsystem
  d_T_m_SG_D_1_block : Subsystem
  d_V_f_SG_D_1_block : Subsystem
  d_psi_1d_SG_D_1_block : Subsystem
  d_psi_d_SG_D_1_block : Subsystem
  d_psi_fd_SG_D_1_block : Subsystem
  d_psi_gq_SG_D_1_block : Subsystem
  d_psi_kq_SG_D_1_block : Subsystem
  d_psi_q_SG_D_1_block : Subsystem
  d_theta_SG_D_1_block : Subsystem
  d_w_SG_D_1_block : Subsystem
  i_d_SG_D_1_block : Subsystem
  i_q_SG_D_1_block : Subsystem
  psi_1d_SG_D_1 : Integrator  InitialCondition=0.8798375031928872
  psi_d_SG_D_1 : Integrator  InitialCondition=0.8530199204188432
  psi_fd_SG_D_1 : Integrator  InitialCondition=1.014998120374068
  psi_gq_SG_D_1 : Integrator  InitialCondition=0.3219550268258626
  psi_kq_SG_D_1 : Integrator  InitialCondition=-0.5030547294154103
  psi_q_SG_D_1 : Integrator  InitialCondition=-0.5231769185920268
  theta_SG_D_1 : Integrator  InitialCondition=0.5498899060731836
  theta_SG_D_1_out_block : Subsystem
  w_SG_D_1 : Integrator  InitialCondition=376.99111843077515
  w_SG_D_1_out_block : Subsystem
  i_d_SG_D_1 : Outport
  i_q_SG_D_1 : Outport  Port=2
  T_e_SG_D_1 : Outport  Port=3
  w_SG_D_1_out : Outport  Port=4
  theta_SG_D_1_out : Outport  Port=5
  wires:
  d_Px_1_SG_D_1_block/1(Blockout_d_Px_1_SG_D_1_0615f) -> Px_1_SG_D_1/1
  V_f_SG_D_1/1 -> d_V_f_SG_D_1_block/14(State_V_f_SG_D_1_44f81), d_E_fd_SG_D_1_block/2(State_V_f_SG_D_1_13d9b)
  psi_kq_SG_D_1/1 -> d_psi_q_SG_D_1_block/2(State_psi_kq_SG_D_1_59706), d_psi_gq_SG_D_1_block/5(State_psi_kq_SG_D_1_b08a9), d_psi_kq_SG_D_1_block/2(State_psi_kq_SG_D_1_0796b), d_w_SG_D_1_block/5(State_psi_kq_SG_D_1_40c17), d_psi_kq_SG_D_1_block/4(State_psi_kq_SG_D_1_e206f), d_psi_gq_SG_D_1_block/8(State_psi_kq_SG_D_1_2559d), i_d_SG_D_1_block/2(State_psi_kq_SG_D_1_e0108), d_psi_gq_SG_D_1_block/3(State_psi_kq_SG_D_1_c7a6a), i_q_SG_D_1_block/2(State_psi_kq_SG_D_1_a7435), d_V_f_SG_D_1_block/10(State_psi_kq_SG_D_1_0096d), T_e_SG_D_1_block/3(State_psi_kq_SG_D_1_0f8e3)
  w_SG_D_1_out_block/1(Blockout_w_SG_D_1_out_bc596) -> w_SG_D_1_out/1
  d_theta_SG_D_1_block/1(Blockout_d_theta_SG_D_1_90efe) -> theta_SG_D_1/1
  w_SG_D_1/1 -> d_psi_d_SG_D_1_block/9(State_w_SG_D_1_b9cd2), d_psi_q_SG_D_1_block/9(State_w_SG_D_1_c3b6c), d_w_SG_D_1_block/1(State_w_SG_D_1_9ad37), d_V_f_SG_D_1_block/8(State_w_SG_D_1_e4672), d_V_f_SG_D_1_block/13(State_w_SG_D_1_348f1), d_T_m_SG_D_1_block/1(State_w_SG_D_1_3ea60), d_theta_SG_D_1_block/1(State_w_SG_D_1_0521f), d_Px_2_SG_D_1_block/4(State_w_SG_D_1_2ac36), d_Px_3_SG_D_1_block/6(State_w_SG_D_1_3feaa), w_SG_D_1_out_block/1(State_w_SG_D_1_b0bc1), d_Px_1_SG_D_1_block/2(State_w_SG_D_1_eeef3)
  d_Px_2_SG_D_1_block/1(Blockout_d_Px_2_SG_D_1_ff825) -> Px_2_SG_D_1/1
  d_T_m_SG_D_1_block/1(Blockout_d_T_m_SG_D_1_63317) -> T_m_SG_D_1/1
  d_Px_3_SG_D_1_block/1(Blockout_d_Px_3_SG_D_1_10237) -> Px_3_SG_D_1/1
  psi_gq_SG_D_1/1 -> d_psi_q_SG_D_1_block/1(State_psi_gq_SG_D_1_ab6b9), d_psi_gq_SG_D_1_block/1(State_psi_gq_SG_D_1_3b3cb), d_psi_gq_SG_D_1_block/4(State_psi_gq_SG_D_1_9bd82), d_psi_gq_SG_D_1_block/2(State_psi_gq_SG_D_1_47aaa), d_psi_kq_SG_D_1_block/1(State_psi_gq_SG_D_1_a2f76), d_psi_kq_SG_D_1_block/3(State_psi_gq_SG_D_1_98e41), d_psi_gq_SG_D_1_block/7(State_psi_gq_SG_D_1_8e432), d_w_SG_D_1_block/4(State_psi_gq_SG_D_1_feebf), d_V_f_SG_D_1_block/9(State_psi_gq_SG_D_1_25411), i_d_SG_D_1_block/1(State_psi_gq_SG_D_1_23547), i_q_SG_D_1_block/1(State_psi_gq_SG_D_1_a3576), T_e_SG_D_1_block/2(State_psi_gq_SG_D_1_d9ca3)
  psi_fd_SG_D_1/1 -> d_psi_fd_SG_D_1_block/10(State_psi_fd_SG_D_1_89e25), d_psi_fd_SG_D_1_block/2(State_psi_fd_SG_D_1_b5722), d_psi_fd_SG_D_1_block/4(State_psi_fd_SG_D_1_7d84c), d_w_SG_D_1_block/10(State_psi_fd_SG_D_1_6a505), i_d_SG_D_1_block/7(State_psi_fd_SG_D_1_b7d62), d_V_f_SG_D_1_block/6(State_psi_fd_SG_D_1_2a3f3), d_psi_1d_SG_D_1_block/2(State_psi_fd_SG_D_1_811e7), d_psi_d_SG_D_1_block/3(State_psi_fd_SG_D_1_3739e), d_psi_fd_SG_D_1_block/7(State_psi_fd_SG_D_1_1d7b9), i_q_SG_D_1_block/7(State_psi_fd_SG_D_1_87227), d_psi_1d_SG_D_1_block/5(State_psi_fd_SG_D_1_382e7), T_e_SG_D_1_block/8(State_psi_fd_SG_D_1_d1c10)
  theta_SG_D_1/1 -> d_psi_d_SG_D_1_block/5(State_theta_SG_D_1_3bf9e), d_psi_d_SG_D_1_block/7(State_theta_SG_D_1_fa062), d_psi_q_SG_D_1_block/5(State_theta_SG_D_1_d9d3f), d_psi_q_SG_D_1_block/7(State_theta_SG_D_1_9a223), i_q_SG_D_1_block/8(State_theta_SG_D_1_18b66), i_d_SG_D_1_block/8(State_theta_SG_D_1_ed7ba), i_d_SG_D_1_block/4(State_theta_SG_D_1_3d426), theta_SG_D_1_out_block/1(State_theta_SG_D_1_cf04f), i_q_SG_D_1_block/4(State_theta_SG_D_1_21b86)
  v_d_SG_D_1/1 -> d_psi_d_SG_D_1_block/4(Input_v_d_SG_D_1_e3573), d_psi_q_SG_D_1_block/4(Input_v_d_SG_D_1_0ed7f)
  v_q_SG_D_1/1 -> d_psi_q_SG_D_1_block/6(Input_v_q_SG_D_1_06492), d_psi_d_SG_D_1_block/6(Input_v_q_SG_D_1_43df0)
  psi_d_SG_D_1/1 -> d_psi_fd_SG_D_1_block/6(State_psi_d_SG_D_1_0c526), d_psi_fd_SG_D_1_block/9(State_psi_d_SG_D_1_a9e00), d_psi_d_SG_D_1_block/2(State_psi_d_SG_D_1_74963), d_psi_q_SG_D_1_block/8(State_psi_d_SG_D_1_bfedb), d_psi_1d_SG_D_1_block/4(State_psi_d_SG_D_1_f98fe), d_w_SG_D_1_block/9(State_psi_d_SG_D_1_3dcbe), d_V_f_SG_D_1_block/12(State_psi_d_SG_D_1_4eb39), i_d_SG_D_1_block/6(State_psi_d_SG_D_1_4d404), i_q_SG_D_1_block/6(State_psi_d_SG_D_1_f2988), d_w_SG_D_1_block/3(State_psi_d_SG_D_1_0b686), T_e_SG_D_1_block/1(State_psi_d_SG_D_1_e2ff8), d_V_f_SG_D_1_block/5(State_psi_d_SG_D_1_4405f), T_e_SG_D_1_block/7(State_psi_d_SG_D_1_8592d)
  Px_1_SG_D_1/1 -> d_Px_1_SG_D_1_block/1(State_Px_1_SG_D_1_dc6c6), d_Px_2_SG_D_1_block/2(State_Px_1_SG_D_1_60b9a), d_Px_3_SG_D_1_block/4(State_Px_1_SG_D_1_9c2b8), d_Px_2_SG_D_1_block/3(State_Px_1_SG_D_1_da658), d_Px_3_SG_D_1_block/5(State_Px_1_SG_D_1_097d2)
  psi_q_SG_D_1/1 -> d_psi_d_SG_D_1_block/8(State_psi_q_SG_D_1_12fad), d_psi_q_SG_D_1_block/3(State_psi_q_SG_D_1_a6dfc), d_psi_gq_SG_D_1_block/6(State_psi_q_SG_D_1_2053d), d_psi_gq_SG_D_1_block/9(State_psi_q_SG_D_1_da7d5), d_psi_kq_SG_D_1_block/5(State_psi_q_SG_D_1_2866b), d_w_SG_D_1_block/6(State_psi_q_SG_D_1_0907a), d_w_SG_D_1_block/7(State_psi_q_SG_D_1_4e93a), d_V_f_SG_D_1_block/11(State_psi_q_SG_D_1_e5350), i_q_SG_D_1_block/3(State_psi_q_SG_D_1_d8456), T_e_SG_D_1_block/4(State_psi_q_SG_D_1_2f227), d_V_f_SG_D_1_block/7(State_psi_q_SG_D_1_08261), T_e_SG_D_1_block/5(State_psi_q_SG_D_1_52964), i_d_SG_D_1_block/3(State_psi_q_SG_D_1_a1fdb)
  Px_2_SG_D_1/1 -> d_Px_2_SG_D_1_block/1(State_Px_2_SG_D_1_69c24), d_Px_3_SG_D_1_block/2(State_Px_2_SG_D_1_a88ed), d_Px_3_SG_D_1_block/3(State_Px_2_SG_D_1_521c0)
  T_m_SG_D_1/1 -> d_T_m_SG_D_1_block/2(State_T_m_SG_D_1_5ba5d), d_w_SG_D_1_block/2(State_T_m_SG_D_1_78758)
  d_E_fd_SG_D_1_block/1(Blockout_d_E_fd_SG_D_1_37355) -> E_fd_SG_D_1/1
  psi_1d_SG_D_1/1 -> d_psi_fd_SG_D_1_block/3(State_psi_1d_SG_D_1_8a938), d_psi_fd_SG_D_1_block/8(State_psi_1d_SG_D_1_69199), d_psi_d_SG_D_1_block/1(State_psi_1d_SG_D_1_18a6b), d_w_SG_D_1_block/8(State_psi_1d_SG_D_1_a2903), d_V_f_SG_D_1_block/4(State_psi_1d_SG_D_1_3e994), i_q_SG_D_1_block/5(State_psi_1d_SG_D_1_a52dc), i_d_SG_D_1_block/5(State_psi_1d_SG_D_1_bbdd2), d_psi_1d_SG_D_1_block/1(State_psi_1d_SG_D_1_4a698), T_e_SG_D_1_block/6(State_psi_1d_SG_D_1_f309e), d_psi_1d_SG_D_1_block/3(State_psi_1d_SG_D_1_ea100), d_psi_fd_SG_D_1_block/5(State_psi_1d_SG_D_1_49865)
  d_V_f_SG_D_1_block/1(Blockout_d_V_f_SG_D_1_81b73) -> V_f_SG_D_1/1
  i_d_SG_D_1_block/1(Blockout_i_d_SG_D_1_69b6a) -> i_d_SG_D_1/1
  d_psi_d_SG_D_1_block/1(Blockout_d_psi_d_SG_D_1_543a6) -> psi_d_SG_D_1/1
  i_q_SG_D_1_block/1(Blockout_i_q_SG_D_1_048b9) -> i_q_SG_D_1/1
  theta_SG_D_1_out_block/1(Blockout_theta_SG_D_1_out_53391) -> theta_SG_D_1_out/1
  d_psi_q_SG_D_1_block/1(Blockout_d_psi_q_SG_D_1_6a810) -> psi_q_SG_D_1/1
  d_psi_kq_SG_D_1_block/1(Blockout_d_psi_kq_SG_D_1_a926e) -> psi_kq_SG_D_1/1
  T_e_SG_D_1_block/1(Blockout_T_e_SG_D_1_2bf50) -> T_e_SG_D_1/1
  d_psi_gq_SG_D_1_block/1(Blockout_d_psi_gq_SG_D_1_db982) -> psi_gq_SG_D_1/1
  d_psi_1d_SG_D_1_block/1(Blockout_d_psi_1d_SG_D_1_96faa) -> psi_1d_SG_D_1/1
  d_R_f_SG_D_1_block/1(Blockout_d_R_f_SG_D_1_5dd2e) -> R_f_SG_D_1/1
  d_w_SG_D_1_block/1(Blockout_d_w_SG_D_1_734e0) -> w_SG_D_1/1
  Px_3_SG_D_1/1 -> d_V_f_SG_D_1_block/3(State_Px_3_SG_D_1_3f381), d_Px_3_SG_D_1_block/1(State_Px_3_SG_D_1_4b68a)
  R_f_SG_D_1/1 -> d_R_f_SG_D_1_block/2(State_R_f_SG_D_1_dba0c), d_V_f_SG_D_1_block/2(State_R_f_SG_D_1_7d9b0)
  E_fd_SG_D_1/1 -> d_V_f_SG_D_1_block/1(State_E_fd_SG_D_1_03212), d_E_fd_SG_D_1_block/1(State_E_fd_SG_D_1_82de9), d_psi_fd_SG_D_1_block/1(State_E_fd_SG_D_1_b74bf), d_R_f_SG_D_1_block/1(State_E_fd_SG_D_1_af68a)
  d_psi_fd_SG_D_1_block/1(Blockout_d_psi_fd_SG_D_1_80960) -> psi_fd_SG_D_1/1
